simulink model "Simulink_21_IOFL"  (R2022b)
settings: Solver=VariableStepAuto  StartTime=0.0  StopTime=10.0  RelTol=1e-3
libraries: simulink x1
settings Model: Creator=a100142  LastModifiedBy=a100142

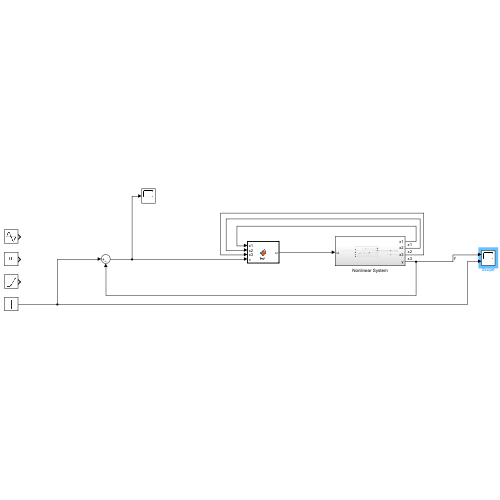
[thumbnail: Simulink's stored preview of the top-level diagram]
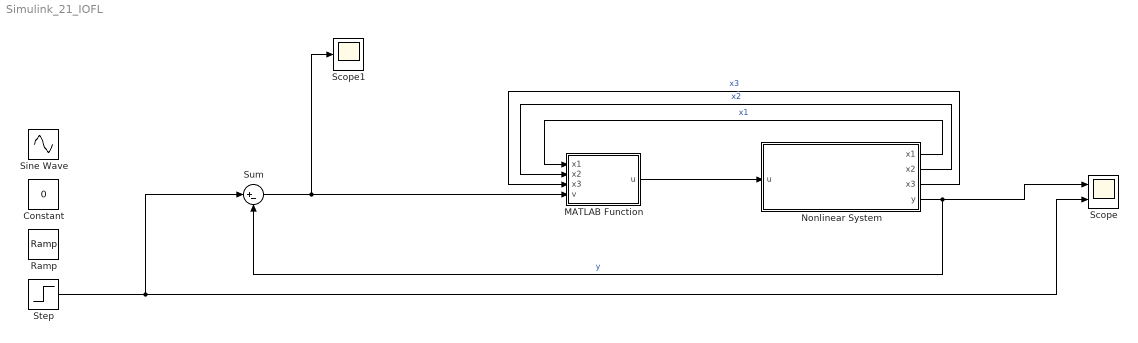
== system Simulink_21_IOFL ==
  Constant : Constant  Value=0
  MATLAB Function : MATLAB Function  TreatAsAtomicUnit=on
  Nonlinear System : Subsystem
  Ramp : simulink/Sources/Ramp  slope=1  start=0  InitialOutput=0
  Scope : Scope  NumInputPorts=2
  Scope1 : Scope
  Sine Wave : Sin  SampleTime=0
  Step : Step  SampleTime=0
  Sum : Sum  Inputs=|+-
  wires:
  MATLAB Function/1(u) -> Nonlinear System/1(u)
  Nonlinear System/1(x1) -> MATLAB Function/1(x1)  "x1"
  Nonlinear System/2(x2) -> MATLAB Function/2(x2)  "x2"
  Nonlinear System/3(x3) -> MATLAB Function/3(x3)  "x3"
  Nonlinear System/4(y) -> Sum/2, Scope/1  "y"
  Sum/1 -> Scope1/1, MATLAB Function/4(v)
  Step/1 -> Sum/1, Scope/2

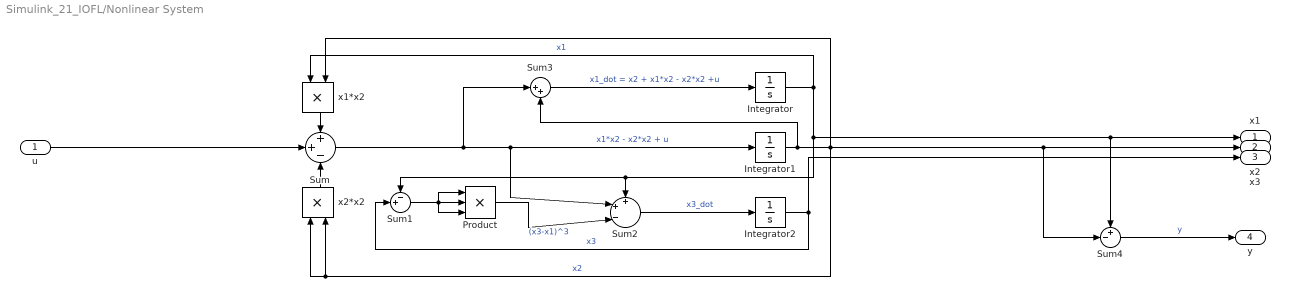
== system Simulink_21_IOFL/Nonlinear System ==
  u : Inport
  Integrator : Integrator  InitialCondition=1
  Integrator1 : Integrator  InitialCondition=1
  Integrator2 : Integrator  InitialCondition=1
  Product : Product  Inputs=3
  Sum : Sum  Inputs=++-
  Sum1 : Sum  Inputs=-+|
  Sum2 : Sum  Inputs=++-|
  Sum3 : Sum  Inputs=|++
  Sum4 : Sum  Inputs=+-|
  x1*x2 : Product
  x2*x2 : Product
  x1 : Outport
  x2 : Outport  Port=2
  x3 : Outport  Port=3
  y : Outport  Port=4
  wires:
  Sum3/1 -> Integrator/1  "x1_dot = x2 + x1*x2 - x2*x2 +u"
  Sum/1 -> Sum3/1, Integrator1/1, Sum2/2  "x1*x2 - x2*x2 + u"
  Product/1 -> Sum2/3  "(x3-x1)^3"
  Integrator/1 -> x1/1, Sum4/1, Sum1/1, Sum2/1, x1*x2/1  "x1"
  Integrator1/1 -> Sum4/2, x2/1, x2*x2/2, x2*x2/1, x1*x2/2, Sum3/2  "x2"
  x2*x2/1 -> Sum/3
  Integrator2/1 -> x3/1, Sum1/2  "x3"
  Sum1/1 -> Product/3, Product/2, Product/1
  x1*x2/1 -> Sum/1
  Sum2/1 -> Integrator2/1  "x3_dot"
  u/1 -> Sum/2
  Sum4/1 -> y/1  "y"

== matlab function Simulink_21_IOFL/MATLAB Function ==
  data: x1 input; u output; x2 input; x3 input; v input
function u = fcn(x1,x2,x3,v)
h = x1-x2;
Lfh = x2;
Lf2h = - x2^2 + x1*x2;
LgLfh = 1;

u =  (v-Lf2h-1.5*Lfh-0.5*h)/LgLfh;
